simulink library "myLibrary"  (R2023b)
settings: Solver=VariableStepAuto  StartTime=0.0  StopTime=10.0  RelTol=1e-3
undefined symbols (not defined in the file): Cac_n1, ctrl1, Da, delta_slk, Discrete, dtha, ee_sli_rtmsupport, FA, gcbh, Ha, Ini, init_DCline, init_IPC, init_line, init_load, init_SG, init_shunt, init_TH, init_trafo, init_user, init_VSC, initMachineBlocks, Ka, Lf, Llkd_pu, Llkq1_pu, magnitude, NET, P, plots_step, q0, Rac_n1, Radd, Rkd_pu, Rkq1_pu, Rload_add, sim_config, sps_rtmsupport, spsSteamTurbineModel, T_DC_NET, T_global, T_IPC, T_load, T_NET, T_SG, T_shunt, T_STATCOM, T_TH, T_trafo, T_user, T_VSC, Ts, tstep, Udiff_a, V1
libraries: spsSeriesRLCBranchLib x120, eeGeneralControl x83, $bdroot x78, spsCurrentMeasurementLib x53, spsParallelRLCBranchLib x39, spsVoltageMeasurementLib x37, spsControlledVoltageSourceLib x30, simulink x29, spsFirstOrderFilterLib x18, spsMeasurementModel x13, spsThreePhaseVIMeasurementLib x5, dspsigops x4
(part 9 of 16)

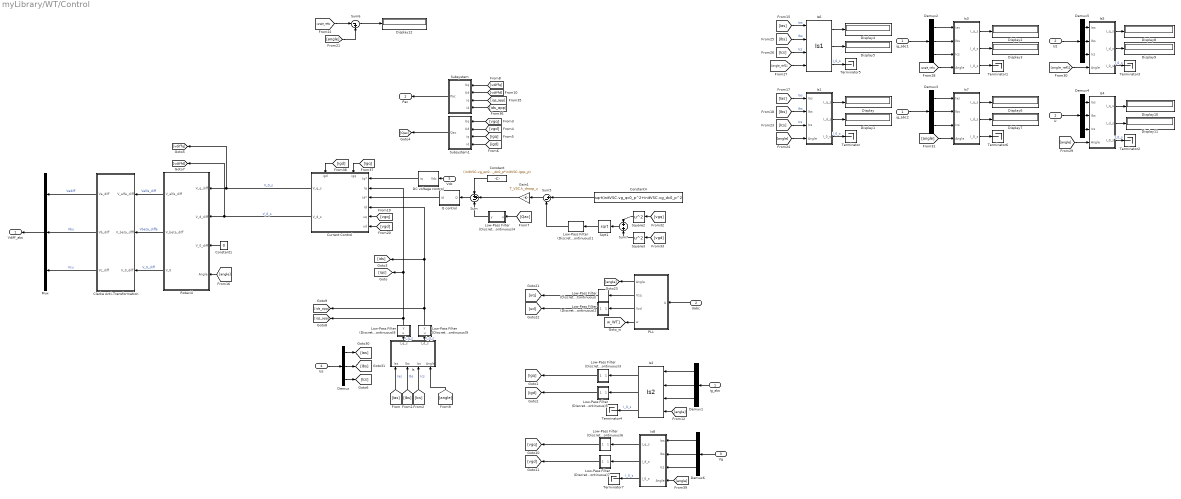
== system myLibrary/WT/Control ==
  ig_abc : Inport
  U : Inport  Port=2
  Vg : Inport  Port=3
  Iss : Inport  Port=4
  Vdc : Inport  Port=5
  Clarke Anti-Transformation : Subsystem
  Constant : Constant  Value=(initVSC.vg_qc0_p*initVSC.igdc_p - initVSC.vg_dc0_p*initVSC.igqc_p)
  Constant1 : Constant  Value=0
  Constant4 : Constant  Value=sqrt(initVSC.vg_qc0_p^2+initVSC.vg_dc0_p^2)
  Current Control : Subsystem
      settings: PortSchema="{\"entries\":[{\"content\":{\"sides\":[{\"content\":{\"connectorIds\":[\"In1\",\"In2\",\"In3\",\"In4\",\"In5\",\"In6\"]},\"type\":\"ConnectorPlacement.EquallySpacedRectSide\",\"uuid\":\"62d33d26-5446-4fb3-9904-ae725dce28a3\"},{\"content\":{\"connectorIds\":[\"Out1\",\"Out2\"],\"side\":\"RIGHT\"},\"type\":\"ConnectorPlacement.EquallySpacedRectSide\",\"uuid\":\"69e0f029-203a-40be-b2c8-c7685bd7a9c9\"},{\"content\":{\"connectorIds\":[\"In7\",\"In8\"],\"side\":\"TOP\"},\"type\":\"ConnectorPlacement.EquallySpacedRectSide\",\"uuid\":\"1d84ed5f-5f23-469b-a3eb-6b4c36cd7918\"}]},\"type\":\"ConnectorPlacement.EquallySpacedConnector\",\"uuid\":\"43257923-4ff4-43c2-a7fb-446a2e70263d\"}],\"packageUris\":[\"http://schema.mathworks.com/mf0/Connector/R2020b\"],\"version\":\"1.0\"}"
  DC voltage control : Subsystem
  Demux{,1..6} (7 alike) : Demux  Outputs=3
  Display{,1..12} (13 alike) : Display
  Gain1 : Gain  Gain=T_VSC.k_droop_u
  Is : Subsystem
  Is1 : Subsystem
  Is2 : $bdroot/GFOR/Control/Is2  SystemSampleTime=-1  VariantActivationTime=update diagram  AllowFlexibleInterface=on  Latency=0  AutoFrameSizeCalculation=off
  Is3 : Subsystem
  Is4 : Subsystem
  Is5 : Subsystem
  Is6 : $bdroot/GFOL/Control/Is1  SystemSampleTime=-1  VariantActivationTime=update diagram  AllowFlexibleInterface=on  Latency=0  AutoFrameSizeCalculation=off
  Is7 : Subsystem
  Is8 : Subsystem
  Low-Pass Filter (Discrete or Continuous) : eeGeneralControl/Low-Pass Filter (Discrete or Continuous)  K=1  T=0  B=inf  A=-inf  init_option=Specify as parameter  x0=initVSC.uqc_p  Ts=-1
  Low-Pass Filter (Discrete or Continuous)1 : eeGeneralControl/Low-Pass Filter (Discrete or Continuous)  K=1  T=T_VSC.tau_droop_u  B=inf  A=-inf  init_option=Specify as parameter  x0=sqrt(initVSC.vg_qc0_p^2+initVSC.vg_dc0_p^2)  Ts=-1
  Low-Pass Filter (Discrete or Continuous)2 : Subsystem  LoadFcn=ee_sli_rtmsupport( 'loadfcn', gcbh );  mask(Low-Pass Filter (Discrete or Continuous)){K=1, T=0, B=inf, A=-inf, init_option=Specify as parameter, x0=initVSC.udc_p, Ts=-1}
      mask prompts: K "physmod:ee:library:comments:control:eeGeneralControl:Gain_MP"; T "physmod:ee:library:comments:control:eeGeneralControl:TimeConstant_MP"; B "physmod:ee:library:comments:control:eeGeneralControl:UpperSaturationLimit_MP"; A "physmod:ee:library:comments:control:eeGeneralControl:LowerSaturationLimit_MP"; init_option "physmod:ee:library:comments:control:eeGeneralControl:Initialization_MP"; x0 "physmod:ee:library:comments:control:eeGeneralControl:InitialState_MP"; Ts "physmod:ee:library:comments:control:eeGeneralControl:SampleTime1ForInherited_MP"
      mask help: physmod:ee:library:comments:control:eeGeneralControl:LowPassFilterDiscreteOrContinuous_MD
      mask init:
      | timeDomain = ee.mask.initializeLowPassFilter(T,B,A,Ts);
      | 
      | ee.mask.callbackPopupInitialization(gcb);
      settings: CopyFcn=ee_sli_rtmsupport( 'copyfcn', gcbh );  DeleteFcn=ee_sli_rtmsupport( 'deletefcn', gcbh );  ModelCloseFcn=ee_sli_rtmsupport( 'modelclosefcn', gcbh );  PostSaveFcn=ee_sli_rtmsupport( 'postsavefcn', gcbh );  PreCopyFcn=ee_sli_rtmsupport( 'precopyfcn', gcbh );  OpenFcn=ee_sli_rtmsupport( 'openfcn', gcbh );  CloseFcn=ee_sli_rtmsupport( 'closefcn', gcbh );  PreDeleteFcn=ee_sli_rtmsupport( 'predeletefcn', gcbh );
      settings: LibrarySourceBlock=|
      | ee_sl_lib/General Control/Low-Pass Filter
      | (Discrete or Continuous)
      mask Help: web(nesl_help(gcbh))
      mask TypeOptions init_option: physmod:ee:library:comments:control:eeGeneralControl:InheritedFromBlockInput_PV | physmod:ee:library:comments:control:eeGeneralControl:SpecifyAsParameter_PV
      mask Callback init_option: ee.mask.callbackPopupInitialization(gcb);
      mask TypeOptions Ts:
      | Integrator
      | (Discrete or Continuous)/Ts
      mask DialogControl ParameterGroupVar Prompt: physmod:ee:library:comments:control:eeGeneralControl:tab_Parameters
      mask DialogControl K Prompt: Gain
      mask DialogControl T Prompt: Time constant
      mask DialogControl B Prompt: Upper saturation limit
      mask DialogControl A Prompt: Lower saturation limit
      mask DialogControl init_option Prompt: Initialization
      mask DialogControl x0 Prompt: Initial state
      mask DialogControl Ts Prompt: Sample time (-1 for inherited)
      mask Display: ee.mask.drawLowPassFilter;
  Low-Pass Filter (Discrete or Continuous)3 : Subsystem  LoadFcn=ee_sli_rtmsupport( 'loadfcn', gcbh );  mask(Low-Pass Filter (Discrete or Continuous)){K=1, T=0, B=inf, A=-inf, init_option=Specify as parameter, x0=initVSC.igqc_p, Ts=-1}
      mask prompts: K "physmod:ee:library:comments:control:eeGeneralControl:Gain_MP"; T "physmod:ee:library:comments:control:eeGeneralControl:TimeConstant_MP"; B "physmod:ee:library:comments:control:eeGeneralControl:UpperSaturationLimit_MP"; A "physmod:ee:library:comments:control:eeGeneralControl:LowerSaturationLimit_MP"; init_option "physmod:ee:library:comments:control:eeGeneralControl:Initialization_MP"; x0 "physmod:ee:library:comments:control:eeGeneralControl:InitialState_MP"; Ts "physmod:ee:library:comments:control:eeGeneralControl:SampleTime1ForInherited_MP"
      mask help: physmod:ee:library:comments:control:eeGeneralControl:LowPassFilterDiscreteOrContinuous_MD
      mask init:
      | timeDomain = ee.mask.initializeLowPassFilter(T,B,A,Ts);
      | 
      | ee.mask.callbackPopupInitialization(gcb);
      settings: CopyFcn=ee_sli_rtmsupport( 'copyfcn', gcbh );  DeleteFcn=ee_sli_rtmsupport( 'deletefcn', gcbh );  ModelCloseFcn=ee_sli_rtmsupport( 'modelclosefcn', gcbh );  PostSaveFcn=ee_sli_rtmsupport( 'postsavefcn', gcbh );  PreCopyFcn=ee_sli_rtmsupport( 'precopyfcn', gcbh );  OpenFcn=ee_sli_rtmsupport( 'openfcn', gcbh );  CloseFcn=ee_sli_rtmsupport( 'closefcn', gcbh );  PreDeleteFcn=ee_sli_rtmsupport( 'predeletefcn', gcbh );
      settings: LibrarySourceBlock=|
      | ee_sl_lib/General Control/Low-Pass Filter
      | (Discrete or Continuous)
      mask Help: web(nesl_help(gcbh))
      mask TypeOptions init_option: physmod:ee:library:comments:control:eeGeneralControl:InheritedFromBlockInput_PV | physmod:ee:library:comments:control:eeGeneralControl:SpecifyAsParameter_PV
      mask Callback init_option: ee.mask.callbackPopupInitialization(gcb);
      mask TypeOptions Ts:
      | Integrator
      | (Discrete or Continuous)/Ts
      mask DialogControl ParameterGroupVar Prompt: physmod:ee:library:comments:control:eeGeneralControl:tab_Parameters
      mask DialogControl K Prompt: Gain
      mask DialogControl T Prompt: Time constant
      mask DialogControl B Prompt: Upper saturation limit
      mask DialogControl A Prompt: Lower saturation limit
      mask DialogControl init_option Prompt: Initialization
      mask DialogControl x0 Prompt: Initial state
      mask DialogControl Ts Prompt: Sample time (-1 for inherited)
      mask Display: ee.mask.drawLowPassFilter;
  Low-Pass Filter (Discrete or Continuous)4 : Subsystem  LoadFcn=ee_sli_rtmsupport( 'loadfcn', gcbh );  mask(Low-Pass Filter (Discrete or Continuous)){K=1, T=T_VSC.tau_droop_u, B=inf, A=-inf, init_option=Specify as parameter, x0=(initVSC.vg_qc0_p*initVSC.igdc_p - initVSC.vg_dc0_p*initVSC.igqc_p), Ts=-1}
      mask prompts: K "physmod:ee:library:comments:control:eeGeneralControl:Gain_MP"; T "physmod:ee:library:comments:control:eeGeneralControl:TimeConstant_MP"; B "physmod:ee:library:comments:control:eeGeneralControl:UpperSaturationLimit_MP"; A "physmod:ee:library:comments:control:eeGeneralControl:LowerSaturationLimit_MP"; init_option "physmod:ee:library:comments:control:eeGeneralControl:Initialization_MP"; x0 "physmod:ee:library:comments:control:eeGeneralControl:InitialState_MP"; Ts "physmod:ee:library:comments:control:eeGeneralControl:SampleTime1ForInherited_MP"
      mask help: physmod:ee:library:comments:control:eeGeneralControl:LowPassFilterDiscreteOrContinuous_MD
      mask init:
      | timeDomain = ee.mask.initializeLowPassFilter(T,B,A,Ts);
      | 
      | ee.mask.callbackPopupInitialization(gcb);
      settings: CopyFcn=ee_sli_rtmsupport( 'copyfcn', gcbh );  DeleteFcn=ee_sli_rtmsupport( 'deletefcn', gcbh );  ModelCloseFcn=ee_sli_rtmsupport( 'modelclosefcn', gcbh );  PostSaveFcn=ee_sli_rtmsupport( 'postsavefcn', gcbh );  PreCopyFcn=ee_sli_rtmsupport( 'precopyfcn', gcbh );  OpenFcn=ee_sli_rtmsupport( 'openfcn', gcbh );  CloseFcn=ee_sli_rtmsupport( 'closefcn', gcbh );  PreDeleteFcn=ee_sli_rtmsupport( 'predeletefcn', gcbh );
      settings: LibrarySourceBlock=|
      | eeGeneralControl/Low-Pass Filter
      | (Discrete or Continuous)
      mask Help: web(nesl_help(gcbh))
      mask TypeOptions init_option: physmod:ee:library:comments:control:eeGeneralControl:InheritedFromBlockInput_PV | physmod:ee:library:comments:control:eeGeneralControl:SpecifyAsParameter_PV
      mask Callback init_option: ee.mask.callbackPopupInitialization(gcb);
      mask TypeOptions Ts:
      | Integrator
      | (Discrete or Continuous)/Ts
      mask DialogControl ParameterGroupVar Prompt: physmod:ee:library:comments:control:eeGeneralControl:tab_Parameters
      mask DialogControl K Prompt: Gain
      mask DialogControl T Prompt: Time constant
      mask DialogControl B Prompt: Upper saturation limit
      mask DialogControl A Prompt: Lower saturation limit
      mask DialogControl init_option Prompt: Initialization
      mask DialogControl x0 Prompt: Initial state
      mask DialogControl Ts Prompt: Sample time (-1 for inherited)
      mask Display: ee.mask.drawLowPassFilter;
  Low-Pass Filter (Discrete or Continuous)5 : Subsystem  LoadFcn=ee_sli_rtmsupport( 'loadfcn', gcbh );  mask(Low-Pass Filter (Discrete or Continuous)){K=1, T=0, B=inf, A=-inf, init_option=Specify as parameter, x0=initVSC.igdc_p, Ts=-1}
      mask prompts: K "physmod:ee:library:comments:control:eeGeneralControl:Gain_MP"; T "physmod:ee:library:comments:control:eeGeneralControl:TimeConstant_MP"; B "physmod:ee:library:comments:control:eeGeneralControl:UpperSaturationLimit_MP"; A "physmod:ee:library:comments:control:eeGeneralControl:LowerSaturationLimit_MP"; init_option "physmod:ee:library:comments:control:eeGeneralControl:Initialization_MP"; x0 "physmod:ee:library:comments:control:eeGeneralControl:InitialState_MP"; Ts "physmod:ee:library:comments:control:eeGeneralControl:SampleTime1ForInherited_MP"
      mask help: physmod:ee:library:comments:control:eeGeneralControl:LowPassFilterDiscreteOrContinuous_MD
      mask init:
      | timeDomain = ee.mask.initializeLowPassFilter(T,B,A,Ts);
      | 
      | ee.mask.callbackPopupInitialization(gcb);
      settings: CopyFcn=ee_sli_rtmsupport( 'copyfcn', gcbh );  DeleteFcn=ee_sli_rtmsupport( 'deletefcn', gcbh );  ModelCloseFcn=ee_sli_rtmsupport( 'modelclosefcn', gcbh );  PostSaveFcn=ee_sli_rtmsupport( 'postsavefcn', gcbh );  PreCopyFcn=ee_sli_rtmsupport( 'precopyfcn', gcbh );  OpenFcn=ee_sli_rtmsupport( 'openfcn', gcbh );  CloseFcn=ee_sli_rtmsupport( 'closefcn', gcbh );  PreDeleteFcn=ee_sli_rtmsupport( 'predeletefcn', gcbh );
      settings: LibrarySourceBlock=|
      | ee_sl_lib/General Control/Low-Pass Filter
      | (Discrete or Continuous)
      mask Help: web(nesl_help(gcbh))
      mask TypeOptions init_option: physmod:ee:library:comments:control:eeGeneralControl:InheritedFromBlockInput_PV | physmod:ee:library:comments:control:eeGeneralControl:SpecifyAsParameter_PV
      mask Callback init_option: ee.mask.callbackPopupInitialization(gcb);
      mask TypeOptions Ts:
      | Integrator
      | (Discrete or Continuous)/Ts
      mask DialogControl ParameterGroupVar Prompt: physmod:ee:library:comments:control:eeGeneralControl:tab_Parameters
      mask DialogControl K Prompt: Gain
      mask DialogControl T Prompt: Time constant
      mask DialogControl B Prompt: Upper saturation limit
      mask DialogControl A Prompt: Lower saturation limit
      mask DialogControl init_option Prompt: Initialization
      mask DialogControl x0 Prompt: Initial state
      mask DialogControl Ts Prompt: Sample time (-1 for inherited)
      mask Display: ee.mask.drawLowPassFilter;
  Low-Pass Filter (Discrete or Continuous)6 : Subsystem  LoadFcn=ee_sli_rtmsupport( 'loadfcn', gcbh );  mask(Low-Pass Filter (Discrete or Continuous)){K=1, T=0, B=inf, A=-inf, init_option=Specify as parameter, x0=initVSC.vg_qc0_p, Ts=-1}
      mask prompts: K "physmod:ee:library:comments:control:eeGeneralControl:Gain_MP"; T "physmod:ee:library:comments:control:eeGeneralControl:TimeConstant_MP"; B "physmod:ee:library:comments:control:eeGeneralControl:UpperSaturationLimit_MP"; A "physmod:ee:library:comments:control:eeGeneralControl:LowerSaturationLimit_MP"; init_option "physmod:ee:library:comments:control:eeGeneralControl:Initialization_MP"; x0 "physmod:ee:library:comments:control:eeGeneralControl:InitialState_MP"; Ts "physmod:ee:library:comments:control:eeGeneralControl:SampleTime1ForInherited_MP"
      mask help: physmod:ee:library:comments:control:eeGeneralControl:LowPassFilterDiscreteOrContinuous_MD
      mask init:
      | timeDomain = ee.mask.initializeLowPassFilter(T,B,A,Ts);
      | 
      | ee.mask.callbackPopupInitialization(gcb);
      settings: CopyFcn=ee_sli_rtmsupport( 'copyfcn', gcbh );  DeleteFcn=ee_sli_rtmsupport( 'deletefcn', gcbh );  ModelCloseFcn=ee_sli_rtmsupport( 'modelclosefcn', gcbh );  PostSaveFcn=ee_sli_rtmsupport( 'postsavefcn', gcbh );  PreCopyFcn=ee_sli_rtmsupport( 'precopyfcn', gcbh );  OpenFcn=ee_sli_rtmsupport( 'openfcn', gcbh );  CloseFcn=ee_sli_rtmsupport( 'closefcn', gcbh );  PreDeleteFcn=ee_sli_rtmsupport( 'predeletefcn', gcbh );
      settings: LibrarySourceBlock=|
      | ee_sl_lib/General Control/Low-Pass Filter
      | (Discrete or Continuous)
      mask Help: web(nesl_help(gcbh))
      mask TypeOptions init_option: physmod:ee:library:comments:control:eeGeneralControl:InheritedFromBlockInput_PV | physmod:ee:library:comments:control:eeGeneralControl:SpecifyAsParameter_PV
      mask Callback init_option: ee.mask.callbackPopupInitialization(gcb);
      mask TypeOptions Ts:
      | Integrator
      | (Discrete or Continuous)/Ts
      mask DialogControl ParameterGroupVar Prompt: physmod:ee:library:comments:control:eeGeneralControl:tab_Parameters
      mask DialogControl K Prompt: Gain
      mask DialogControl T Prompt: Time constant
      mask DialogControl B Prompt: Upper saturation limit
      mask DialogControl A Prompt: Lower saturation limit
      mask DialogControl init_option Prompt: Initialization
      mask DialogControl x0 Prompt: Initial state
      mask DialogControl Ts Prompt: Sample time (-1 for inherited)
      mask Display: ee.mask.drawLowPassFilter;
  Low-Pass Filter (Discrete or Continuous)7 : Subsystem  LoadFcn=ee_sli_rtmsupport( 'loadfcn', gcbh );  mask(Low-Pass Filter (Discrete or Continuous)){K=1, T=0, B=inf, A=-inf, init_option=Specify as parameter, x0=initVSC.vg_dc0_p, Ts=-1}
      mask prompts: K "physmod:ee:library:comments:control:eeGeneralControl:Gain_MP"; T "physmod:ee:library:comments:control:eeGeneralControl:TimeConstant_MP"; B "physmod:ee:library:comments:control:eeGeneralControl:UpperSaturationLimit_MP"; A "physmod:ee:library:comments:control:eeGeneralControl:LowerSaturationLimit_MP"; init_option "physmod:ee:library:comments:control:eeGeneralControl:Initialization_MP"; x0 "physmod:ee:library:comments:control:eeGeneralControl:InitialState_MP"; Ts "physmod:ee:library:comments:control:eeGeneralControl:SampleTime1ForInherited_MP"
      mask help: physmod:ee:library:comments:control:eeGeneralControl:LowPassFilterDiscreteOrContinuous_MD
      mask init:
      | timeDomain = ee.mask.initializeLowPassFilter(T,B,A,Ts);
      | 
      | ee.mask.callbackPopupInitialization(gcb);
      settings: CopyFcn=ee_sli_rtmsupport( 'copyfcn', gcbh );  DeleteFcn=ee_sli_rtmsupport( 'deletefcn', gcbh );  ModelCloseFcn=ee_sli_rtmsupport( 'modelclosefcn', gcbh );  PostSaveFcn=ee_sli_rtmsupport( 'postsavefcn', gcbh );  PreCopyFcn=ee_sli_rtmsupport( 'precopyfcn', gcbh );  OpenFcn=ee_sli_rtmsupport( 'openfcn', gcbh );  CloseFcn=ee_sli_rtmsupport( 'closefcn', gcbh );  PreDeleteFcn=ee_sli_rtmsupport( 'predeletefcn', gcbh );
      settings: LibrarySourceBlock=|
      | ee_sl_lib/General Control/Low-Pass Filter
      | (Discrete or Continuous)
      mask Help: web(nesl_help(gcbh))
      mask TypeOptions init_option: physmod:ee:library:comments:control:eeGeneralControl:InheritedFromBlockInput_PV | physmod:ee:library:comments:control:eeGeneralControl:SpecifyAsParameter_PV
      mask Callback init_option: ee.mask.callbackPopupInitialization(gcb);
      mask TypeOptions Ts:
      | Integrator
      | (Discrete or Continuous)/Ts
      mask DialogControl ParameterGroupVar Prompt: physmod:ee:library:comments:control:eeGeneralControl:tab_Parameters
      mask DialogControl K Prompt: Gain
      mask DialogControl T Prompt: Time constant
      mask DialogControl B Prompt: Upper saturation limit
      mask DialogControl A Prompt: Lower saturation limit
      mask DialogControl init_option Prompt: Initialization
      mask DialogControl x0 Prompt: Initial state
      mask DialogControl Ts Prompt: Sample time (-1 for inherited)
      mask Display: ee.mask.drawLowPassFilter;
  Low-Pass Filter (Discrete or Continuous)8 : Subsystem  LoadFcn=ee_sli_rtmsupport( 'loadfcn', gcbh );  mask(Low-Pass Filter (Discrete or Continuous)){K=1, T=0, B=inf, A=-inf, init_option=Specify as parameter, x0=initVSC.idiffqc_p, Ts=-1}
      mask prompts: K "physmod:ee:library:comments:control:eeGeneralControl:Gain_MP"; T "physmod:ee:library:comments:control:eeGeneralControl:TimeConstant_MP"; B "physmod:ee:library:comments:control:eeGeneralControl:UpperSaturationLimit_MP"; A "physmod:ee:library:comments:control:eeGeneralControl:LowerSaturationLimit_MP"; init_option "physmod:ee:library:comments:control:eeGeneralControl:Initialization_MP"; x0 "physmod:ee:library:comments:control:eeGeneralControl:InitialState_MP"; Ts "physmod:ee:library:comments:control:eeGeneralControl:SampleTime1ForInherited_MP"
      mask help: physmod:ee:library:comments:control:eeGeneralControl:LowPassFilterDiscreteOrContinuous_MD
      mask init:
      | timeDomain = ee.mask.initializeLowPassFilter(T,B,A,Ts);
      | 
      | ee.mask.callbackPopupInitialization(gcb);
      settings: CopyFcn=ee_sli_rtmsupport( 'copyfcn', gcbh );  DeleteFcn=ee_sli_rtmsupport( 'deletefcn', gcbh );  ModelCloseFcn=ee_sli_rtmsupport( 'modelclosefcn', gcbh );  PostSaveFcn=ee_sli_rtmsupport( 'postsavefcn', gcbh );  PreCopyFcn=ee_sli_rtmsupport( 'precopyfcn', gcbh );  OpenFcn=ee_sli_rtmsupport( 'openfcn', gcbh );  CloseFcn=ee_sli_rtmsupport( 'closefcn', gcbh );  PreDeleteFcn=ee_sli_rtmsupport( 'predeletefcn', gcbh );
      settings: LibrarySourceBlock=|
      | ee_sl_lib/General Control/Low-Pass Filter
      | (Discrete or Continuous)
      mask Help: web(nesl_help(gcbh))
      mask TypeOptions init_option: physmod:ee:library:comments:control:eeGeneralControl:InheritedFromBlockInput_PV | physmod:ee:library:comments:control:eeGeneralControl:SpecifyAsParameter_PV
      mask Callback init_option: ee.mask.callbackPopupInitialization(gcb);
      mask TypeOptions Ts:
      | Integrator
      | (Discrete or Continuous)/Ts
      mask DialogControl ParameterGroupVar Prompt: physmod:ee:library:comments:control:eeGeneralControl:tab_Parameters
      mask DialogControl K Prompt: Gain
      mask DialogControl T Prompt: Time constant
      mask DialogControl B Prompt: Upper saturation limit
      mask DialogControl A Prompt: Lower saturation limit
      mask DialogControl init_option Prompt: Initialization
      mask DialogControl x0 Prompt: Initial state
      mask DialogControl Ts Prompt: Sample time (-1 for inherited)
      mask Display: ee.mask.drawLowPassFilter;
  Low-Pass Filter (Discrete or Continuous)9 : Subsystem  LoadFcn=ee_sli_rtmsupport( 'loadfcn', gcbh );  mask(Low-Pass Filter (Discrete or Continuous)){K=1, T=0, B=inf, A=-inf, init_option=Specify as parameter, x0=initVSC.idiffdc_p, Ts=-1}
      mask prompts: K "physmod:ee:library:comments:control:eeGeneralControl:Gain_MP"; T "physmod:ee:library:comments:control:eeGeneralControl:TimeConstant_MP"; B "physmod:ee:library:comments:control:eeGeneralControl:UpperSaturationLimit_MP"; A "physmod:ee:library:comments:control:eeGeneralControl:LowerSaturationLimit_MP"; init_option "physmod:ee:library:comments:control:eeGeneralControl:Initialization_MP"; x0 "physmod:ee:library:comments:control:eeGeneralControl:InitialState_MP"; Ts "physmod:ee:library:comments:control:eeGeneralControl:SampleTime1ForInherited_MP"
      mask help: physmod:ee:library:comments:control:eeGeneralControl:LowPassFilterDiscreteOrContinuous_MD
      mask init:
      | timeDomain = ee.mask.initializeLowPassFilter(T,B,A,Ts);
      | 
      | ee.mask.callbackPopupInitialization(gcb);
      settings: CopyFcn=ee_sli_rtmsupport( 'copyfcn', gcbh );  DeleteFcn=ee_sli_rtmsupport( 'deletefcn', gcbh );  ModelCloseFcn=ee_sli_rtmsupport( 'modelclosefcn', gcbh );  PostSaveFcn=ee_sli_rtmsupport( 'postsavefcn', gcbh );  PreCopyFcn=ee_sli_rtmsupport( 'precopyfcn', gcbh );  OpenFcn=ee_sli_rtmsupport( 'openfcn', gcbh );  CloseFcn=ee_sli_rtmsupport( 'closefcn', gcbh );  PreDeleteFcn=ee_sli_rtmsupport( 'predeletefcn', gcbh );
      settings: LibrarySourceBlock=|
      | ee_sl_lib/General Control/Low-Pass Filter
      | (Discrete or Continuous)
      mask Help: web(nesl_help(gcbh))
      mask TypeOptions init_option: physmod:ee:library:comments:control:eeGeneralControl:InheritedFromBlockInput_PV | physmod:ee:library:comments:control:eeGeneralControl:SpecifyAsParameter_PV
      mask Callback init_option: ee.mask.callbackPopupInitialization(gcb);
      mask TypeOptions Ts:
      | Integrator
      | (Discrete or Continuous)/Ts
      mask DialogControl ParameterGroupVar Prompt: physmod:ee:library:comments:control:eeGeneralControl:tab_Parameters
      mask DialogControl K Prompt: Gain
      mask DialogControl T Prompt: Time constant
      mask DialogControl B Prompt: Upper saturation limit
      mask DialogControl A Prompt: Lower saturation limit
      mask DialogControl init_option Prompt: Initialization
      mask DialogControl x0 Prompt: Initial state
      mask DialogControl Ts Prompt: Sample time (-1 for inherited)
      mask Display: ee.mask.drawLowPassFilter;
  Mux : Mux  Inputs=3
  PLL : Subsystem
  Q control : Subsystem
  Rotació : Subsystem
  Sqrt1 : Sqrt
  Square2 : Math  Operator=square
  Square3 : Math  Operator=square
  Subsystem : Subsystem
  Subsystem1 : Subsystem
  Sum : Sum  Inputs=++-
  Sum5 : Sum  Inputs=|+-
  Sum6 : Sum  Inputs=|-+
  Sum7 : Sum
  Terminator{,1..7} (8 alike) : Terminator
  U2 : InportShadow  Port=2
  Uabc : InportShadow  Port=2
  ig_abc1 : InportShadow
  ig_abc2 : InportShadow
  Vdiff_abc : Outport
  Pac : Outport  Port=2
  tag scope: w_WT1=global
  wires:
  Is2/2 -> Low-Pass Filter (Discrete or Continuous)5/1(u)
  Is2/1 -> Low-Pass Filter (Discrete or Continuous)3/1(u)
  PLL/3(Vzd) -> Low-Pass Filter (Discrete or Continuous)2/1(u)
  PLL/2(Vzq) -> Low-Pass Filter (Discrete or Continuous)/1
  [angle] -> Is7/4(Angle)
  Is7/1(I_q_s) -> Display6/1
  Is7/2(I_d_s) -> Display7/1
  Is7/3(I_0_s) -> Terminator6/1
  Demux3/1 -> Is7/1(Ias)
  Demux3/2 -> Is7/2(Ibs)
  Demux3/3 -> Is7/3(Ics)
  ig_abc2/1 -> Demux3/1
  [Ias] -> Is6/1  "Ias"
  [Ibs] -> Is6/2  "Ibs"
  [Ics] -> Is6/3  "Ics"
  [angle_ref1] -> Is6/4
  Is6/1 -> Display4/1
  Is6/2 -> Display5/1
  Is6/3 -> Terminator5/1  "I_0_s"
  ig_abc1/1 -> Demux2/1
  Demux2/3 -> Is3/3(Ics)
  Demux2/2 -> Is3/2(Ibs)
  Demux2/1 -> Is3/1(Ias)
  Constant1/1 -> Rotació/3(V_0_diff)
  Mux/1 -> Vdiff_abc/1
  Clarke Anti-Transformation/2(Vb_diff) -> Mux/2  "Vbu"
  Clarke Anti-Transformation/3(Vc_diff) -> Mux/3  "Vcu"
  Rotació/3(V_0) -> Clarke Anti-Transformation/3(V_0_diff)  "V_0_diff"
  Clarke Anti-Transformation/1(Va_diff) -> Mux/1  "Vadiff"
  Rotació/2(V_beta_diff) -> Clarke Anti-Transformation/2(V_beta_dfff)  "Vbeta_diffa"
  Rotació/1(V_alfa_diff) -> Clarke Anti-Transformation/1(V_alfa_diff)  "Valfa_diff"
  Is5/3(I_0_s) -> Terminator3/1  "I_0_s"
  Is4/3(I_0_s) -> Terminator2/1  "I_0_s"
  Is3/3(I_0_s) -> Terminator1/1
  Is1/3(I_0_s) -> Terminator/1  "I_0_s"
  Is5/2(I_d_s) -> Display9/1
  Is5/1(I_q_s) -> Display8/1
  Is4/2(I_d_s) -> Display11/1
  Is4/1(I_q_s) -> Display10/1
  Is3/2(I_d_s) -> Display3/1
  Is3/1(I_q_s) -> Display2/1
  Is1/2(I_d_s) -> Display1/1
  Is1/1(I_q_s) -> Display/1
  U2/1 -> Demux5/1
  Demux5/1 -> Is5/1(Ias)
  Demux5/2 -> Is5/2(Ibs)
  Demux5/3 -> Is5/3(Ics)
  [angle_ref1] -> Is5/4(Angle)
  [angle] -> Is4/4(Angle)
  Demux4/3 -> Is4/3(Ics)
  Demux4/2 -> Is4/2(Ibs)
  Demux4/1 -> Is4/1(Ias)
  U/1 -> Demux4/1
  [angle_ref1] -> Is3/4(Angle)
  [angle] -> Is1/4(Angle)
  [Ics] -> Is1/3(Ics)  "Ics"
  [Ibs] -> Is1/2(Ibs)  "Ibs"
  [Ias] -> Is1/1(Ias)  "Ias"
  [angle_ref1] -> Sum6/1
  Sum6/1 -> Display12/1
  [angle] -> Sum6/2
  [vgd] -> Current Control/6(ud)
  [vgq] -> Current Control/5(uq)
  Current Control/2(V_d_s) -> [vdiffd], Rotació/2(V_d_diff)  "V_0_s"
  Current Control/1(V_q_s) -> [vdiffq], Rotació/1(V_q_diff)  "V_0_s"
  [angle] -> Rotació/4(Angle)
  [angle] -> Is/4(Angle)
  Iss/1 -> Demux/1
  Demux/3 -> [Ics]
  Demux/2 -> [Ibs]
  Demux/1 -> [Ias]
  Uabc/1 -> PLL/1(U)
  PLL/1(Angle) -> [angle]
  [Ibs] -> Is/2(Ibs)  "Ibs"
  [Ics] -> Is/3(Ics)  "Ics"
  [Ias] -> Is/1(Ias)  "Ias"
  Is/1(I_q_s) -> Low-Pass Filter (Discrete or Continuous)8/1(u)  "I_q_s"
  Is/2(I_d_s) -> Low-Pass Filter (Discrete or Continuous)9/1(u)  "I_d_s"
  PLL/4(w) -> [w_WT1]
  Demux1/1 -> Is2/1
  Demux1/3 -> Is2/3
  ig_abc/1 -> Demux1/1
  Is2/3 -> Terminator4/1  "I_0_s"
  [angle] -> Is2/4
  Demux1/2 -> Is2/2
  Square3/1 -> Sum7/2
  Low-Pass Filter (Discrete or Continuous)1/1 -> Sum5/2
  [vgq] -> Square2/1
  [vgd] -> Square3/1
  Sqrt1/1 -> Low-Pass Filter (Discrete or Continuous)1/1
  Square2/1 -> Sum7/1
  Sum7/1 -> Sqrt1/1
  Vdc/1 -> DC voltage control/1(Vdc)
  Subsystem/1(Pac) -> Pac/1
  Constant4/1 -> Sum5/1
  Sum5/1 -> Gain1/1
  [igd] -> Subsystem1/4(id)
  [igq] -> Subsystem1/3(iq)
  [vgd] -> Subsystem1/2(Ud)
  [vgq] -> Subsystem1/1(Uq)
  Subsystem1/1(Qac) -> [Qac]
  [Qac] -> Low-Pass Filter (Discrete or Continuous)4/1(u)
  Sum/1 -> Q control/1(Q)
  [vdiffq] -> Subsystem/1(Uq)
  [vdiffd] -> Subsystem/2(Ud)
  [iqs_app] -> Subsystem/3(iq)
  [ids_app] -> Subsystem/4(id)
  Low-Pass Filter (Discrete or Continuous)4/1(y) -> Sum/3
  Gain1/1 -> Sum/2
  Constant/1 -> Sum/1
  Demux6/2 -> Is8/2(Ibs)
  [angle] -> Is8/4(Angle)
  Is8/3(I_0_s) -> Terminator7/1  "I_0_s"
  Vg/1 -> Demux6/1
  Demux6/3 -> Is8/3(Ics)
  Demux6/1 -> Is8/1(Ias)
  Is8/1(I_q_s) -> Low-Pass Filter (Discrete or Continuous)6/1(u)
  Is8/2(I_d_s) -> Low-Pass Filter (Discrete or Continuous)7/1(u)
  [igq] -> Current Control/7(igq)
  [igd] -> Current Control/8(igd)
  DC voltage control/1(iq) -> Current Control/1(Iq*)
  Q control/1(id) -> Current Control/3(Id*)
  Low-Pass Filter (Discrete or Continuous)/1 -> [uq]
  Low-Pass Filter (Discrete or Continuous)2/1(y) -> [ud]
  Low-Pass Filter (Discrete or Continuous)3/1(y) -> [igq]
  Low-Pass Filter (Discrete or Continuous)5/1(y) -> [igd]
  Low-Pass Filter (Discrete or Continuous)6/1(y) -> [vgq]
  Low-Pass Filter (Discrete or Continuous)7/1(y) -> [vgd]
  Low-Pass Filter (Discrete or Continuous)8/1(y) -> [iqs], Current Control/2(Iq), [iqs_app]
  Low-Pass Filter (Discrete or Continuous)9/1(y) -> [ids_app], [ids], Current Control/4(Id)

== system myLibrary/WT/Delay ==
  In1 : Inport
  Transport Delay1 : TransportDelay  DelayTime=T_VSC.tau_cmd  InitialOutput=[initVSC.Udiff_a_delay, initVSC.Udiff_b_delay, initVSC.Udiff_c_delay]  PadeOrder=2
  Unit Delay : UnitDelay  InitialCondition=[initVSC.Udiff_a, initVSC.Udiff_b, initVSC.Udiff_c]  SampleTime=T_VSC.tau_cmd  HasFrameUpgradeWarning=on
  Out1 : Outport
  wires:
  In1/1 -> Transport Delay1/1
  Transport Delay1/1 -> Out1/1

== system myLibrary/WT/Electrical ==
  note: DIFF CIRCUIT:
  Pac : Inport
  vdiff : Inport  Port=2
  Constant : Constant  Value=initVSC.Pdc
  Constant5 : Constant  Value=[ 2/3 1/3; -1/3 1/3 ; -1/3 -2/3]
  Controlled Voltage Source1 : spsControlledVoltageSourceLib/Controlled Voltage Source  Initialize=on  Source_Type=AC  Amplitude=initVSC.Udiff_mag  Phase=initVSC.angle_vdiff*180/pi  Frequency=T_VSC.fb  Measurements=None
  Controlled Voltage Source2 : spsControlledVoltageSourceLib/Controlled Voltage Source  Initialize=on  Source_Type=AC  Amplitude=initVSC.Udiff_mag  Phase=(initVSC.angle_vdiff -2*pi/3)*180/pi  Frequency=T_VSC.fb  Measurements=None
  Controlled Voltage Source3 : spsControlledVoltageSourceLib/Controlled Voltage Source  Initialize=on  Source_Type=AC  Amplitude=initVSC.Udiff_mag  Phase=(initVSC.angle_vdiff +2*pi/3)*180/pi  Frequency=T_VSC.fb  Measurements=None
  Demux : Demux  Outputs=3
  Divide1 : Product  Inputs=*/
  Gain : Gain  Gain=1/T_VSC.Ceq
  Gain1 : Gain  Gain=-1
  Ig_l2g2 : Gain
  Integrator : Integrator  InitialCondition=2*sqrt(3/2)
  Mesura Ias10 : spsCurrentMeasurementLib/Current Measurement  PhasorSimulation=off  OutputType=Complex  PSBequivalent=0
  Mesura Ias7 : spsCurrentMeasurementLib/Current Measurement  PhasorSimulation=off  OutputType=Complex  PSBequivalent=0
  Mesura Ias9 : spsCurrentMeasurementLib/Current Measurement  PhasorSimulation=off  OutputType=Complex  PSBequivalent=0
  Mux : Mux  Inputs=3
  Mux10 : Mux  Inputs=2
  Power7 : Subsystem  DialogController=POWERSYS.PowerSysDialog  LoadFcn=sps_rtmsupport('LoadFcn', gcbh);  StartFcn=sps_rtmsupport('StartFcn', gcbh);  StopFcn=sps_rtmsupport('StopFcn', gcbh);  mask(Power (3ph, Instantaneous)){}
      mask help:
      | Compute the three-phase instantaneous active and reactive powers associated with a periodic set of three-phase voltages and currents.
      |
      | Instantaneous reactive power is accurate only for balanced and harmonic-free three-phase voltages and currents.
      |
      | Current flowing into an RL circuit will produce positive active and reactive power.
      settings: CopyFcn=sps_rtmsupport('CopyFcn', gcbh);  DeleteFcn=sps_rtmsupport('DeleteFcn', gcbh);  UndoDeleteFcn=sps_rtmsupport('UndoDeleteFcn', gcbh);  ModelCloseFcn=sps_rtmsupport('ModelCloseFcn', gcbh);  PreSaveFcn=sps_rtmsupport('PreSaveFcn', gcbh);  PostSaveFcn=sps_rtmsupport('PostSaveFcn', gcbh);  NameChangeFcn=sps_rtmsupport('NameChangeFcn', gcbh);  PreCopyFcn=sps_rtmsupport('PreCopyFcn', gcbh);  OpenFcn=sps_rtmsupport('OpenFcn', gcbh, []);  CloseFcn=sps_rtmsupport('CloseFcn', gcbh);  PreDeleteFcn=sps_rtmsupport('PreDeleteFcn', gcbh);
      settings: LibrarySourceBlock=|
      | spsPower3phInstantaneousLib/Power
      | (3ph, Instantaneous)
      mask Help: helpview(psbhelp);
  Product4 : Product  Multiplication=Matrix(*)
  Sum : Sum  Inputs=|+-
  Terminator : Terminator
  Voltage Measurement : spsVoltageMeasurementLib/Voltage Measurement  PhasorSimulation=off  OutputType=Complex  PSBequivalent=0
  Voltage Measurement1 : Subsystem  DialogController=POWERSYS.PowerSysDialog  LoadFcn=sps_rtmsupport('LoadFcn',gcbh);  StartFcn=sps_rtmsupport('StartFcn',gcbh);  StopFcn=sps_rtmsupport('StopFcn',gcbh);  mask(Voltage Measurement){PhasorSimulation=off, OutputType=Complex, PSBequivalent=0}
      mask prompts: PhasorSimulation "Phasor simulation"; OutputType "Output signal :"; PSBequivalent "Equivalent circuit"
      mask help: Ideal voltage measurement. The Output signal parameter is disabled when the block is not used in a phasor simulation. The phasor simulation is activated by a Powergui block placed in the model.
      mask init: same as myLibrary/HVDC_line/Current Measurement1
      settings: LibrarySourceBlock=sps_lib/Sensors and Measurements/Voltage Measurement  CopyFcn=sps_rtmsupport('CopyFcn',gcbh); powericon('psbloadfunction',gcb,'Measurement Block','UpdateGotoTag');  DeleteFcn=sps_rtmsupport('DeleteFcn',gcbh);  UndoDeleteFcn=sps_rtmsupport('UndoDeleteFcn',gcbh);  ModelCloseFcn=sps_rtmsupport('ModelCloseFcn',gcbh);  PreSaveFcn=sps_rtmsupport('PreSaveFcn',gcbh);  PostSaveFcn=sps_rtmsupport('PostSaveFcn',gcbh);  NameChangeFcn=sps_rtmsupport('NameChangeFcn',gcbh);powericon('SetNewGotoTag',[gcb,'/source'],-2);  PreCopyFcn=sps_rtmsupport('PreCopyFcn',gcbh);  OpenFcn=sps_rtmsupport('OpenFcn',gcbh, [1 -2]);  CloseFcn=sps_rtmsupport('CloseFcn',gcbh);  PreDeleteFcn=sps_rtmsupport('PreDeleteFcn',gcbh);
      mask Help: helpview(psbhelp);
      mask TypeOptions OutputType: Complex | Real-Imag | Magnitude-Angle | Magnitude
  Zsa : spsSeriesRLCBranchLib/Series RLC Branch  LConnTagsString=__new0  RConnTagsString=__new0  BranchType=RL  Resistance=initVSC.Rc  Inductance=initVSC.Lc  SetiL0=off  InitialCurrent=initVSC.Isa  Capacitance=1e-6  Setx0=off  InitialVoltage=0  Measurements=None
  Zsa1 : spsSeriesRLCBranchLib/Series RLC Branch  LConnTagsString=__new0  RConnTagsString=__new0  BranchType=RL  Resistance=initVSC.Rc  Inductance=initVSC.Lc  SetiL0=on  InitialCurrent=initVSC.Isb  Capacitance=1e-6  Setx0=off  InitialVoltage=0  Measurements=None
  Zsa2 : spsSeriesRLCBranchLib/Series RLC Branch  LConnTagsString=__new0  RConnTagsString=__new0  BranchType=RL  Resistance=initVSC.Rc  Inductance=initVSC.Lc  SetiL0=on  InitialCurrent=initVSC.Isc  Capacitance=1e-6  Setx0=off  InitialVoltage=0  Measurements=None
  VA : PMIOPort  Side=Left
  VB : PMIOPort  Port=2  Side=Left
  VC : PMIOPort  Port=3  Side=Left
  Vdc : Outport
  Is : Outport  Port=2
  wires:
  [Vdiffc] -> Controlled Voltage Source3/1
  [Vdiffb] -> Controlled Voltage Source2/1
  [Vdiffa] -> Controlled Voltage Source1/1
  [Ias] -> Mux/1  "Ias"
  [Ibs] -> Mux/2  "Ibs"
  [Ics] -> Mux/3  "Ics"
  Demux/2 -> [Vdiffb]
  Demux/3 -> [Vdiffc]
  Demux/1 -> [Vdiffa]
  vdiff/1 -> Demux/1
  Mesura Ias9/1 -> [Ibs]
  Mesura Ias7/1 -> [Ias]
  Mesura Ias10/1 -> [Ics]
  Pac/1 -> [Pac]
  Integrator/1 -> [Vdc], Divide1/2
  Gain/1 -> Integrator/1
  Divide1/1 -> Gain/1
  Gain1/1 -> Divide1/1
  [Vdc] -> Vdc/1  "Ics"
  [Pac_vsc] -> Sum/1  "Ics"
  Sum/1 -> Gain1/1
  Constant/1 -> Sum/2
  Power7/2(Q) -> Terminator/1
  Ig_l2g2/1 -> [Pac_vsc]
  Power7/1(P) -> Ig_l2g2/1
  Mux/1 -> Is/1, Power7/2(Iabc)
  Mux10/1 -> Product4/2
  Constant5/1 -> Product4/1
  Product4/1 -> Power7/1(Vabc)
  Voltage Measurement/1 -> Mux10/1
  Voltage Measurement1/1(v) -> Mux10/2
  connections:
  Controlled Voltage Source2/LConn1 -- Controlled Voltage Source1/LConn1 -- Controlled Voltage Source3/LConn1
  Zsa2/RConn1 -- Mesura Ias10/LConn1
  Zsa1/RConn1 -- Mesura Ias9/LConn1
  Zsa/RConn1 -- Mesura Ias7/LConn1
  Mesura Ias10/RConn1 -- VC/RConn1
  Mesura Ias9/RConn1 -- VB/RConn1
  Mesura Ias7/RConn1 -- VA/RConn1
  Zsa1/LConn1 -- Voltage Measurement/LConn2 -- Voltage Measurement1/LConn1 -- Controlled Voltage Source2/RConn1
  Zsa2/LConn1 -- Voltage Measurement1/LConn2 -- Controlled Voltage Source3/RConn1
  Zsa/LConn1 -- Voltage Measurement/LConn1 -- Controlled Voltage Source1/RConn1

== system myLibrary/WT/Filter Ig ==
  In1 : Inport
  Second-Order Filter6 : Subsystem  DialogController=POWERSYS.PowerSysDialog  LoadFcn=sps_rtmsupport('LoadFcn', gcbh);  StartFcn=sps_rtmsupport('StartFcn', gcbh);  StopFcn=sps_rtmsupport('StopFcn', gcbh);  mask(Second-Order Filter){FilterType=Lowpass, Fo=T_VSC.fc, Zeta=1/sqrt(2), Ts=0, Initialize=on, Vac_Init=[initVSC.Ig_mag,  initVSC.angle_ig*180/pi,  T_VSC.fb; initVSC.Ig_mag,  initVSC.angle_ig*180/pi-120,  T_VSC.fb; initVSC.Ig_mag,  initVSC.angle_ig*180/pi+120,  T_VSC.fb], Vdc_Init=[0;0;0], PlotResponse=off, FreqRange=[0, 500, 1]}
      mask prompts: FilterType "Filter type:"; Fo "Natural frequency fn (Hz):"; Zeta "Damping ratio Zeta ( Q = 1 / (2*Zeta) ):"; Ts "Sample time:"; Initialize "Initialize filter states"; Vac_Init "AC initial input: [ Mag, Phase (degrees),  Freq (Hz) ]:"; Vdc_Init "DC initial input:"; PlotResponse "Plot filter response"; FreqRange "Frequency range(Hz) [ Start,  End,  Inc.]:"
      mask help: Implement a lowpass, highpass, bandpass, or bandstop second-order filter.
      mask init:
      | block=gcb;
      | [WantBlockChoice,Ts,sps] = powericon('SecondOrderFilterInit',block,FilterType,Fo,Zeta,Initialize,Vac_Init,Vdc_Init,Ts);
      | powericon('SecondOrderFilterInit',FilterType,Fo,Zeta,PlotResponse,FreqRange);
      | powericon('SetInternalModels','set',block,WantBlockChoice);
      settings: CopyFcn=sps_rtmsupport('CopyFcn', gcbh);  DeleteFcn=sps_rtmsupport('DeleteFcn', gcbh);  UndoDeleteFcn=sps_rtmsupport('UndoDeleteFcn', gcbh);  ModelCloseFcn=sps_rtmsupport('ModelCloseFcn', gcbh);  PreSaveFcn=sps_rtmsupport('PreSaveFcn', gcbh);  PostSaveFcn=sps_rtmsupport('PostSaveFcn', gcbh);  NameChangeFcn=sps_rtmsupport('NameChangeFcn', gcbh);  PreCopyFcn=sps_rtmsupport('PreCopyFcn', gcbh);  OpenFcn="sps_rtmsupport('OpenFcn', gcbh, [1  5  8]);"  CloseFcn=sps_rtmsupport('CloseFcn', gcbh);  PreDeleteFcn=sps_rtmsupport('PreDeleteFcn', gcbh);
      settings: LibrarySourceBlock=|
      | sps_lib/Control/Filters/Second-Order
      | Filter
      mask Help: helpview(psbhelp);
      mask TypeOptions FilterType: Lowpass | Highpass | Bandpass | Bandstop (Notch)
      mask Callback Initialize: powericon('SecondOrderFilterInit',gcb);
      mask Callback PlotResponse: powericon('SecondOrderFilterInit',gcb);
      mask Display: plot(sps.X,sps.Y);
  Zero-Order Hold2 : ZeroOrderHold  SampleTime=T_VSC.tau_zoh
  Out1 : Outport
  wires:
  In1/1 -> Second-Order Filter6/1(In)
  Zero-Order Hold2/1 -> Out1/1
  Second-Order Filter6/1(Out) -> Zero-Order Hold2/1

== system myLibrary/WT/Filter Is ==
  In1 : Inport
  Second-Order Filter3 : Subsystem  DialogController=POWERSYS.PowerSysDialog  LoadFcn=sps_rtmsupport('LoadFcn', gcbh);  StartFcn=sps_rtmsupport('StartFcn', gcbh);  StopFcn=sps_rtmsupport('StopFcn', gcbh);  mask(Second-Order Filter){FilterType=Lowpass, Fo=T_VSC.fc, Zeta=1/sqrt(2), Ts=0, Initialize=on, Vac_Init=[initVSC.Is_mag,  initVSC.angle_is*180/pi,  T_VSC.fb; initVSC.Is_mag,  initVSC.angle_is*180/pi-120,  T_VSC.fb;initVSC.Is_mag,  initVSC.angle_is*180/pi+120,  T_VSC.fb], Vdc_Init=[0;0;0], PlotResponse=off, FreqRange=[0, 500, 1]}
      mask prompts: FilterType "Filter type:"; Fo "Natural frequency fn (Hz):"; Zeta "Damping ratio Zeta ( Q = 1 / (2*Zeta) ):"; Ts "Sample time:"; Initialize "Initialize filter states"; Vac_Init "AC initial input: [ Mag, Phase (degrees),  Freq (Hz) ]:"; Vdc_Init "DC initial input:"; PlotResponse "Plot filter response"; FreqRange "Frequency range(Hz) [ Start,  End,  Inc.]:"
      mask help: Implement a lowpass, highpass, bandpass, or bandstop second-order filter.
      mask init: same as myLibrary/WT/Filter Ig/Second-Order Filter6
      settings: CopyFcn=sps_rtmsupport('CopyFcn', gcbh);  DeleteFcn=sps_rtmsupport('DeleteFcn', gcbh);  UndoDeleteFcn=sps_rtmsupport('UndoDeleteFcn', gcbh);  ModelCloseFcn=sps_rtmsupport('ModelCloseFcn', gcbh);  PreSaveFcn=sps_rtmsupport('PreSaveFcn', gcbh);  PostSaveFcn=sps_rtmsupport('PostSaveFcn', gcbh);  NameChangeFcn=sps_rtmsupport('NameChangeFcn', gcbh);  PreCopyFcn=sps_rtmsupport('PreCopyFcn', gcbh);  OpenFcn="sps_rtmsupport('OpenFcn', gcbh, [1  5  8]);"  CloseFcn=sps_rtmsupport('CloseFcn', gcbh);  PreDeleteFcn=sps_rtmsupport('PreDeleteFcn', gcbh);
      settings: LibrarySourceBlock=|
      | sps_lib/Control/Filters/Second-Order
      | Filter
      mask Help: helpview(psbhelp);
      mask TypeOptions FilterType: Lowpass | Highpass | Bandpass | Bandstop (Notch)
      mask Callback Initialize: powericon('SecondOrderFilterInit',gcb);
      mask Callback PlotResponse: powericon('SecondOrderFilterInit',gcb);
      mask Display: plot(sps.X,sps.Y);
  Zero-Order Hold4 : ZeroOrderHold  SampleTime=T_VSC.tau_zoh
  Out1 : Outport
  wires:
  In1/1 -> Second-Order Filter3/1(In)
  Second-Order Filter3/1(Out) -> Zero-Order Hold4/1
  Zero-Order Hold4/1 -> Out1/1

== system myLibrary/WT/Filter U ==
  In1 : Inport
  Demux : Demux  Commented=on  Outputs=3
  Demux1 : Demux  Commented=on  Outputs=3
  Demux2 : Demux  Commented=on  Outputs=3
  Gain : Gain  Commented=on
  Integrator : Integrator  Commented=on
  Scope : Scope  Commented=on  NumInputPorts=2
  Scope1 : Scope  Commented=on  NumInputPorts=2
  Second-Order Filter6 : $bdroot/WT/Filter Ig/Second-Order Filter6  FilterType=Lowpass  Fo=T_VSC.fc  Zeta=1/sqrt(2)  Ts=0  Initialize=on  Vac_Init="[initVSC.U_mag,  initVSC.angle_umag*180/pi,  T_VSC.fb; initVSC.U_mag,  initVSC.angle_umag*180/pi-120,  T_VSC.fb; initVSC.U_mag,  initVSC.angle_umag*180/pi+120,  T_VSC.fb]"  Vdc_Init=[0;0;0]  PlotResponse=off  FreqRange=[0, 500, 1]
      settings: LibrarySourceBlock=|
      | sps_lib/Control/Filters/Second-Order
      | Filter
  Sum : Sum  Commented=on  Inputs=|-+
  Transport Delay1 : TransportDelay  Commented=on  DelayTime=T_VSC.tau_zoh  PadeOrder=2
  Zero-Order Hold5 : ZeroOrderHold  SampleTime=T_VSC.tau_zoh
  Out1 : Outport
  wires:
  In1/1 -> Second-Order Filter6/1
  Second-Order Filter6/1 -> Gain/1, Transport Delay1/1, Demux/1, Zero-Order Hold5/1
  Zero-Order Hold5/1 -> Demux1/1, Out1/1
  Demux/1 -> Scope1/1, Scope/1
  Demux1/1 -> Scope/2
  Demux2/1 -> Scope1/2
  Transport Delay1/1 -> Sum/1
  Gain/1 -> Sum/2
  Sum/1 -> Integrator/1
  Integrator/1 -> Demux2/1

== system myLibrary/WT/Filter Vdc ==
  In1 : Inport
  Second-Order Filter1 : Subsystem  DialogController=POWERSYS.PowerSysDialog  LoadFcn=sps_rtmsupport('LoadFcn', gcbh);  StartFcn=sps_rtmsupport('StartFcn', gcbh);  StopFcn=sps_rtmsupport('StopFcn', gcbh);  mask(Second-Order Filter){FilterType=Lowpass, Fo=T_VSC.fc, Zeta=1/sqrt(2), Ts=0, Initialize=on, Vac_Init=[0,  0,  0], Vdc_Init=2, PlotResponse=off, FreqRange=[0, 500, 1]}
      mask prompts: FilterType "Filter type:"; Fo "Natural frequency fn (Hz):"; Zeta "Damping ratio Zeta ( Q = 1 / (2*Zeta) ):"; Ts "Sample time:"; Initialize "Initialize filter states"; Vac_Init "AC initial input: [ Mag, Phase (degrees),  Freq (Hz) ]:"; Vdc_Init "DC initial input:"; PlotResponse "Plot filter response"; FreqRange "Frequency range(Hz) [ Start,  End,  Inc.]:"
      mask help: Implement a lowpass, highpass, bandpass, or bandstop second-order filter.
      mask init: same as myLibrary/WT/Filter Ig/Second-Order Filter6
      settings: CopyFcn=sps_rtmsupport('CopyFcn', gcbh);  DeleteFcn=sps_rtmsupport('DeleteFcn', gcbh);  UndoDeleteFcn=sps_rtmsupport('UndoDeleteFcn', gcbh);  ModelCloseFcn=sps_rtmsupport('ModelCloseFcn', gcbh);  PreSaveFcn=sps_rtmsupport('PreSaveFcn', gcbh);  PostSaveFcn=sps_rtmsupport('PostSaveFcn', gcbh);  NameChangeFcn=sps_rtmsupport('NameChangeFcn', gcbh);  PreCopyFcn=sps_rtmsupport('PreCopyFcn', gcbh);  OpenFcn="sps_rtmsupport('OpenFcn', gcbh, [1  5  8]);"  CloseFcn=sps_rtmsupport('CloseFcn', gcbh);  PreDeleteFcn=sps_rtmsupport('PreDeleteFcn', gcbh);
      settings: LibrarySourceBlock=|
      | sps_lib/Control/Filters/Second-Order
      | Filter
      mask Help: helpview(psbhelp);
      mask TypeOptions FilterType: Lowpass | Highpass | Bandpass | Bandstop (Notch)
      mask Callback Initialize: powericon('SecondOrderFilterInit',gcb);
      mask Callback PlotResponse: powericon('SecondOrderFilterInit',gcb);
      mask Display: plot(sps.X,sps.Y);
  Zero-Order Hold1 : ZeroOrderHold  SampleTime=T_VSC.tau_zoh
  Out1 : Outport
  wires:
  In1/1 -> Second-Order Filter1/1(In)
  Second-Order Filter1/1(Out) -> Zero-Order Hold1/1
  Zero-Order Hold1/1 -> Out1/1

== system myLibrary/WT/Filter Vg ==
  In1 : Inport
  Second-Order Filter6 : $bdroot/WT/Filter Ig/Second-Order Filter6  FilterType=Lowpass  Fo=T_VSC.fc  Zeta=1/sqrt(2)  Ts=0  Initialize=on  Vac_Init="[initVSC.Vg_mag,  initVSC.angle_vg*180/pi,  T_VSC.fb; initVSC.Vg_mag,  initVSC.angle_vg*180/pi-120,  T_VSC.fb; initVSC.Vg_mag,  initVSC.angle_vg*180/pi+120,  T_VSC.fb]"  Vdc_Init=[0;0;0]  PlotResponse=off  FreqRange=[0, 500, 1]
      settings: LibrarySourceBlock=|
      | sps_lib/Control/Filters/Second-Order
      | Filter
  Zero-Order Hold3 : ZeroOrderHold  SampleTime=T_VSC.tau_zoh
  Out1 : Outport
  wires:
  In1/1 -> Second-Order Filter6/1
  Zero-Order Hold3/1 -> Out1/1
  Second-Order Filter6/1 -> Zero-Order Hold3/1

== system myLibrary/qd transform/qd0 Transformation ==
  a : Inport
  b : Inport  Port=2
  c : Inport  Port=3
  Angle : Inport  Port=4
  Demux1 : Demux  Outputs=3
  Matriu T : Subsystem
  Mux : Mux  Inputs=3
  Product : Product  Multiplication=Matrix(*)
  Terminator : Terminator
  q : Outport  VectorParamsAs1DForOutWhenUnconnected=off
  d : Outport  Port=2  VectorParamsAs1DForOutWhenUnconnected=off
  wires:
  Product/1 -> Demux1/1
  Matriu T/1(Out1) -> Product/1
  Demux1/1 -> q/1
  Demux1/2 -> d/1
  Demux1/3 -> Terminator/1
  Angle/1 -> Matriu T/1(u)
  Mux/1 -> Product/2
  a/1 -> Mux/1
  b/1 -> Mux/2
  c/1 -> Mux/3

== system myLibrary/AC-GFOL_DC-GFOL/Control Pac2/Calcul Energies2 ==
  Vs : Inport
  Demux : Demux  Outputs=6
  Gain{1..6} (6 alike) : Gain  Gain=T_IPC.Carm/2
  Math Function{1..6} (6 alike) : Math  Operator=magnitude^2  SignedPower=on
  Sum4 : Sum  Inputs=|++
  Sum5 : Sum  Inputs=|++
  Sum9 : Sum  Inputs=|++
  Eat : Outport
  Ebt : Outport  Port=2
  Ect : Outport  Port=3
  wires:
  [Ebl] -> Sum5/2
  Gain5/1 -> [Ecu]  "Ecu"
  [Eau] -> Sum4/1
  Gain1/1 -> [Eau]  "Eau"
  Gain2/1 -> [Eal]  "Eal"
  [Ecu] -> Sum9/1
  Math Function4/1 -> Gain4/1
  [Ecl] -> Sum9/2
  Math Function1/1 -> Gain1/1
  Gain4/1 -> [Ebl]  "Ebl"
  [Ebu] -> Sum5/1
  Gain6/1 -> [Ecl]  "Ecl"
  Sum9/1 -> Ect/1
  Math Function5/1 -> Gain5/1
  [Vcls] -> Math Function6/1
  Math Function2/1 -> Gain2/1
  [Vbus] -> Math Function3/1
  Sum5/1 -> Ebt/1
  Math Function6/1 -> Gain6/1
  [Vals] -> Math Function2/1
  [Vaus] -> Math Function1/1
  Math Function3/1 -> Gain3/1
  Sum4/1 -> Eat/1
  Gain3/1 -> [Ebu]  "Ebu"
  [Eal] -> Sum4/2
  [Vcus] -> Math Function5/1
  [Vbls] -> Math Function4/1
  Vs/1 -> Demux/1
  Demux/1 -> [Vaus]
  Demux/2 -> [Vals]
  Demux/3 -> [Vbus]
  Demux/4 -> [Vbls]
  Demux/5 -> [Vcus]
  Demux/6 -> [Vcls]

== system myLibrary/AC-GFOL_DC-GFOL/Control Pac2/Clarke Anti-Transformation ==
  V_alfa_diff : Inport
  V_beta_dfff : Inport  Port=2
  V_0_diff : Inport  Port=3
  Constant{,2,5,8} (4 alike) : Constant
  Constant1 : Constant  Value=0
  Constant3 : Constant  Value=-1/2
  Constant4 : Constant  Value=-sqrt(3)/2
  Constant6 : Constant  Value=-1/2
  Constant7 : Constant  Value=sqrt(3)/2
  Demux : Demux  Outputs=3
  Display : Display
  Math Function : Math  Operator=transpose  SignedPower=on
  Matrix Concatenate : Concatenate  NumInputs=3  Mode=Multidimensional array  ConcatenateDimension=2
  Mux{,1..3} (4 alike) : Mux  Inputs=3
  Product : Product  Multiplication=Matrix(*)
  Va_diff : Outport  VectorParamsAs1DForOutWhenUnconnected=off
  Vb_diff : Outport  Port=2  VectorParamsAs1DForOutWhenUnconnected=off
  Vc_diff : Outport  Port=3  VectorParamsAs1DForOutWhenUnconnected=off
  wires:
  Constant/1 -> Mux1/1
  Constant1/1 -> Mux1/2
  Constant2/1 -> Mux1/3
  Constant3/1 -> Mux2/1
  Constant4/1 -> Mux2/2
  Constant5/1 -> Mux2/3
  Constant6/1 -> Mux3/1
  Constant7/1 -> Mux3/2
  Constant8/1 -> Mux3/3
  Matrix Concatenate/1 -> Math Function/1
  Mux2/1 -> Matrix Concatenate/2
  Mux3/1 -> Matrix Concatenate/3
  Mux1/1 -> Matrix Concatenate/1
  Product/1 -> Demux/1
  Demux/1 -> Va_diff/1  "Va"
  Demux/2 -> Vb_diff/1  "Vb"
  Demux/3 -> Vc_diff/1  "Vc"
  Mux/1 -> Product/2
  Math Function/1 -> Display/1, Product/1
  V_alfa_diff/1 -> Mux/1  "Valfa"
  V_beta_dfff/1 -> Mux/2  "Vbeta"
  V_0_diff/1 -> Mux/3  "0"
